simulink model "Demo919"  (R2018b)
settings: Solver=ode3  StartTime=0.0  StopTime=10  FixedStep=0.0005  RelTol=1e-3  EnableMultiTasking=on
values from neighbouring files (symbols this model uses):
  ADS1 = [1000 4000]    [data_new1.m]
  ADS2 = [900 4100]    [data_new1.m]
  br_opening = [0 20 40 60 80 100]    [data_new1.m]
  BRAKE = [485 1288 2091 2894 3697 4500]    [data_new1.m]
  InerWheel_Angle = [0 0.001 0.502 1.006 1.514 2.024 2.538 3.055 3.575 4.098 4.625 5.155 5.689 6.226 6.767 7.311 7.859 8.411 8.967 9.527 10.091 10.659 11.231 11.807 12.387 12.972 13.561 14.154 14.752 15.354 15.961 16.572 17.187 17.807 18.432 19.062 19.696 20.334 20.977 21.625 22.277 22.934 23.596 24.262 24.932 25.607 26.286 26.970 27.657 28.349 29.045 29.745 30.448 31.155 31.866]    [data_new1.m]
  OuterWheel_Angle = [0 0.001 0.501 1.001 1.501 2.001 2.501	3.001 3.501	4.001 4.501	5.001 5.501	6.001 6.501	7.001 7.501	8.001 8.501	9.001 9.501	10.001 10.501 11.001 11.501 12.001 12.501 13.001 13.501	14.001 14.501 15.001 15.501 16.001 16.501 17.001 17.501 18.001 18.501 19.001 19.501	20.001 20.501 21.001 21.501	22.001 22.501 23.001 23.501	24.001 24.501 25.001 25.501 26.001 26.501]    [data_new1.m]
  PUMP = [0 1000 2000 3000 4000 5000]    [data_new1.m]
  SteeringAngle_Cal = [-90 0 90]    [data_new1.m]
  SteeringAngle_Sensor = [640 1840 3041]    [data_new1.m]
  th_opening = [0 100]    [data_new1.m]
undefined symbols (not defined in the file or in its folder): D, I_AN06_5V, I_AN08_5V, I_AN09_5V, I_AN10_5V, I_HALL1, I_HALL2, I_SW01_L, I_SW10_L, I_SW11_H, I_SW12_H, I_SW13_H, I_SW14_H, I_SW15_H, I_SW16_H, I_SW17_H, I_SW18_H, I_SW19_H, I_SW20_H, O_PWM1_LS0A7, O_PWM2_LS0A7, O_SW02_LS0A4, O_SW13_HS1A, O_SW14_HS1A
libraries: ec5744lib x137, simulink x20, canmsglib x11
(part 2 of 5)

== system Demo919/Function-Call Subsystem1/Subsystem ==
  note: 油压范围在500到4500之间
  note: 输出12V高电平给蜂鸣器和待驶指示
      | 灯，启动鸣笛，指示灯亮
  Brake : Inport  OutDataTypeStr=uint16
  Key : Inport  Port=2
  MCU1_rdy : Inport  Port=3
  MCU2_rdy : Inport  Port=4
  DC_BusVoltH1 : Inport  Port=5
  DC_BusVoltL1 : Inport  Port=6
  DC_BusVoltH2 : Inport  Port=7
  DC_BusVoltL2 : Inport  Port=8
  1-D Lookup Table2 : Lookup_n-D  NumberOfTableDimensions=1  BreakpointsForDimension1=BRAKE  Table=br_opening  ExtrapMethod=Clip  InternalRulePriority=Speed  OutMin=0  OutMax=100  OutDataTypeStr=uint8  RndMeth=Simplest  InputSameDT=on
  MeaModule : ec5744lib/RapidECU_U3/07Calibration/MeaModule  signal=Wait_Start
      settings: SourceProductName=ECUCoder for MPC5744
  MeaModule1 : ec5744lib/RapidECU_U3/07Calibration/MeaModule  signal=Brake
      settings: SourceProductName=ECUCoder for MPC5744
  MeaModule2 : ec5744lib/RapidECU_U3/07Calibration/MeaModule  signal=brake
      settings: SourceProductName=ECUCoder for MPC5744
  MeaModule3 : ec5744lib/RapidECU_U3/07Calibration/MeaModule  signal=RS
      settings: SourceProductName=ECUCoder for MPC5744
  Subsystem1 : Subsystem
  Subsystem2 : Subsystem
  Terminator : Terminator
  WaitStart&Brake_LED : Stateflow chart  TreatAsAtomicUnit=on
  "Brake " : Outport
  Break_LED : Outport  Port=2
  WS_Sig : Outport  Port=3
  Wait_Start : Outport  Port=4
  wires:
  WaitStart&Brake_LED/1(Wait_Start) -> MeaModule/1  "Wait_Start"
  Brake/1 -> MeaModule2/1
  1-D Lookup Table2/1 -> "Brake "/1, MeaModule1/1
  WaitStart&Brake_LED/2(Break_LED) -> Break_LED/1  "Break_LED"
  Key/1 -> WaitStart&Brake_LED/2(Key)
  WaitStart&Brake_LED/3(WS_Sig) -> WS_Sig/1
  WaitStart&Brake_LED/4(RS) -> MeaModule3/1
  MeaModule3/1 -> Terminator/1
  MCU1_rdy/1 -> WaitStart&Brake_LED/3(MCU1_rdy)
  MCU2_rdy/1 -> WaitStart&Brake_LED/4(MCU2_rdy)
  MeaModule/1 -> Wait_Start/1
  DC_BusVoltH1/1 -> Subsystem1/1(DatH)
  DC_BusVoltL1/1 -> Subsystem1/2(DatL)
  DC_BusVoltH2/1 -> Subsystem2/1(DatH)
  DC_BusVoltL2/1 -> Subsystem2/2(DatL)
  Subsystem1/1(DC_BusVolt1) -> WaitStart&Brake_LED/5(DC_BusVolt1)
  Subsystem2/1(DC_BusVolt2) -> WaitStart&Brake_LED/6(DC_BusVolt2)
  MeaModule1/1 -> WaitStart&Brake_LED/1(Brake)
  MeaModule2/1 -> 1-D Lookup Table2/1

== system Demo919/Function-Call Subsystem1/Subsystem1 ==
  Re_Mot_Speed : Inport
  Add : Sum  AccumDataTypeStr=double
  Add1 : Sum  AccumDataTypeStr=double
  Add2 : Sum  Inputs=-+
  Add3 : Sum  Inputs=+-
  Bus Creator : BusCreator  Inputs=2
  Bus Selector : BusSelector  OutputSignals=Re_Mot_SpeedL1,Re_Mot_SpeedH1,Re_Mot_SpeedL2,Re_Mot_SpeedH2
  Constant : Constant  Value=10000
  Constant1 : Constant  Value=10000
  Data Type Conversion{,1..3} (4 alike) : DataTypeConversion  OutDataTypeStr=uint16
  Data Type Conversion6 : DataTypeConversion  OutDataTypeStr=double
  Data Type Conversion7 : DataTypeConversion  OutDataTypeStr=double
  Gain : Gain  Gain=0.5
  Gain1 : Gain  Gain=0.5
  Shift Arithmetic : ArithShift  BitShiftNumber=8  BitShiftDirection=Left
  Shift Arithmetic1 : ArithShift  BitShiftNumber=8  BitShiftDirection=Left
  Mot_Speed : Outport
  wires:
  Bus Selector/3 -> Data Type Conversion2/1  "<Re_Mot_SpeedL2>"
  Bus Selector/1 -> Data Type Conversion/1  "<Re_Mot_SpeedL1>"
  Bus Selector/2 -> Data Type Conversion1/1  "<Re_Mot_SpeedH1>"
  Re_Mot_Speed/1 -> Bus Selector/1
  Bus Selector/4 -> Data Type Conversion3/1  "<Re_Mot_SpeedH2>"
  Data Type Conversion6/1 -> Gain/1
  Data Type Conversion7/1 -> Gain1/1
  Constant1/1 -> Add3/2
  Constant/1 -> Add2/1
  Add3/1 -> Bus Creator/2
  Gain1/1 -> Add3/1
  Add2/1 -> Bus Creator/1
  Gain/1 -> Add2/2
  Bus Creator/1 -> Mot_Speed/1
  Data Type Conversion3/1 -> Shift Arithmetic1/1
  Add1/1 -> Data Type Conversion7/1
  Data Type Conversion2/1 -> Add1/1
  Shift Arithmetic1/1 -> Add1/2
  Add/1 -> Data Type Conversion6/1
  Shift Arithmetic/1 -> Add/2
  Data Type Conversion1/1 -> Shift Arithmetic/1
  Data Type Conversion/1 -> Add/1

== system Demo919/Function-Call Subsystem1/Subsystem2 ==
  Bus_Curr&Volt : Inport
  Abs : Abs
  Bus Selector6 : BusSelector  OutputSignals=Bat_Voltage_MSB,Bat_Voltage_LSB,Bat_Current_MSB,Bat_Current_LSB
  Gain : Gain  Gain=1/1000
  Product : Product
  Subsystem4 : Subsystem
  Subsystem5 : Subsystem
  P : Outport
  wires:
  Bus_Curr&Volt/1 -> Bus Selector6/1
  Gain/1 -> Abs/1
  Bus Selector6/1 -> Subsystem4/1(CurrH)  "<Bat_Voltage_MSB>"
  Bus Selector6/2 -> Subsystem4/2(CurrL)  "<Bat_Voltage_LSB>"
  Bus Selector6/3 -> Subsystem5/1(CurrH)  "<Bat_Current_MSB>"
  Bus Selector6/4 -> Subsystem5/2(CurrL)  "<Bat_Current_LSB>"
  Subsystem4/1(Bat_V) -> Product/1
  Subsystem5/1(Bat_A) -> Product/2
  Abs/1 -> P/1
  Product/1 -> Gain/1

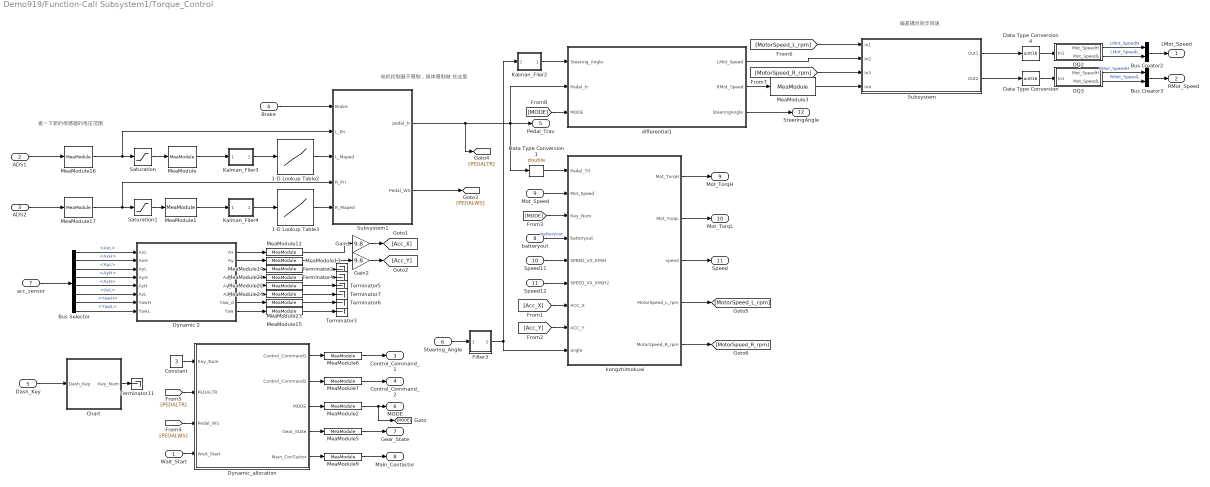
== system Demo919/Function-Call Subsystem1/Torque_Control ==
  note: 偏差耦合同步转速
  note: 查一下新的传感器的电压范围
  note: 电机控制器不限制，具体限制做
      | 在这里
  Wait_Start : Inport
  ADS1 : Inport  Port=2
  ADS2 : Inport  Port=3  OutDataTypeStr=uint16
  "Brake " : Inport  Port=4
  "Dash_Key " : Inport  Port=5  OutMin=0  OutMax=2
  Steering_Angle : Inport  Port=6
  acc_sensor : Inport  Port=7
  batteryout : Inport  Port=8
  Mot_Speed : Inport  Port=9
  Speed11 : Inport  Port=10
  Speed12 : Inport  Port=11
  1-D Lookup Table2 : Lookup_n-D  NumberOfTableDimensions=1  BreakpointsForDimension1=ADS1  Table=th_opening  ExtrapMethod=Clip  InternalRulePriority=Speed  OutMin=0  OutMax=95  OutDataTypeStr=double  RndMeth=Simplest  InputSameDT=on
  1-D Lookup Table3 : Lookup_n-D  NumberOfTableDimensions=1  BreakpointsForDimension1=ADS2  Table=th_opening  ExtrapMethod=Clip  InternalRulePriority=Speed  OutMin=0  OutMax=95  OutDataTypeStr=double  RndMeth=Simplest  InputSameDT=on
  Bus Creator2 : BusCreator  Inputs=2
  Bus Creator3 : BusCreator  Inputs=2
  Bus Selector : BusSelector  OutputSignals=AxL,AxH,AyL,AyH,AzH,AzL,YawH,YawL
  Chart : Stateflow chart  TreatAsAtomicUnit=on
  Constant : Constant  Value=3
  Data Type Conversion : DataTypeConversion  OutDataTypeStr=uint16
  Data Type Conversion1 : DataTypeConversion  OutDataTypeStr=double
  Data Type Conversion4 : DataTypeConversion  OutDataTypeStr=uint16
  Dynamic 2 : Stateflow chart  TreatAsAtomicUnit=on
  Dynamic_allocation : Stateflow chart  TreatAsAtomicUnit=on
  Filter3 : Subsystem
  Gain1 : Gain  Gain=9.8
  Gain2 : Gain  Gain=9.8
  Kalman_Filer2 : Subsystem
  Kalman_Filer3 : Subsystem
  Kalman_Filer4 : Subsystem
  MeaModule : ec5744lib/RapidECU_U3/07Calibration/MeaModule  signal=ADSH
      settings: SourceProductName=ECUCoder for MPC5744
  MeaModule1 : ec5744lib/RapidECU_U3/07Calibration/MeaModule  signal=ADSL
      settings: SourceProductName=ECUCoder for MPC5744
  MeaModule12 : ec5744lib/RapidECU_U3/07Calibration/MeaModule  signal=AX
      settings: SourceProductName=ECUCoder for MPC5744
  MeaModule13 : ec5744lib/RapidECU_U3/07Calibration/MeaModule  signal=AY
      settings: SourceProductName=ECUCoder for MPC5744
  MeaModule14 : ec5744lib/RapidECU_U3/07Calibration/MeaModule  signal=AZ
      settings: SourceProductName=ECUCoder for MPC5744
  MeaModule15 : ec5744lib/RapidECU_U3/07Calibration/MeaModule  signal=YAW
      settings: SourceProductName=ECUCoder for MPC5744
  MeaModule16 : ec5744lib/RapidECU_U3/07Calibration/MeaModule  signal=ADSh
      settings: SourceProductName=ECUCoder for MPC5744
  MeaModule17 : ec5744lib/RapidECU_U3/07Calibration/MeaModule  signal=ADSl
      settings: SourceProductName=ECUCoder for MPC5744
  MeaModule2 : ec5744lib/RapidECU_U3/07Calibration/MeaModule  signal=MODE
      settings: SourceProductName=ECUCoder for MPC5744
  MeaModule21 : ec5744lib/RapidECU_U3/07Calibration/MeaModule  signal=Ax_d
      settings: SourceProductName=ECUCoder for MPC5744
  MeaModule22 : ec5744lib/RapidECU_U3/07Calibration/MeaModule  signal=Ay_d
      settings: SourceProductName=ECUCoder for MPC5744
  MeaModule23 : ec5744lib/RapidECU_U3/07Calibration/MeaModule  signal=Yaw_d
      settings: SourceProductName=ECUCoder for MPC5744
  MeaModule24 : ec5744lib/RapidECU_U3/07Calibration/MeaModule  signal=Az_d
      settings: SourceProductName=ECUCoder for MPC5744
  MeaModule3 : ec5744lib/RapidECU_U3/07Calibration/MeaModule  signal=RMotSpeed
      settings: SourceProductName=ECUCoder for MPC5744
  MeaModule5 : ec5744lib/RapidECU_U3/07Calibration/MeaModule  signal=Gear_State
      settings: SourceProductName=ECUCoder for MPC5744
  MeaModule6 : ec5744lib/RapidECU_U3/07Calibration/MeaModule  signal=Control1
      settings: SourceProductName=ECUCoder for MPC5744
  MeaModule7 : ec5744lib/RapidECU_U3/07Calibration/MeaModule  signal=Control2
      settings: SourceProductName=ECUCoder for MPC5744
  MeaModule9 : ec5744lib/RapidECU_U3/07Calibration/MeaModule  signal=Main_Contactor
      settings: SourceProductName=ECUCoder for MPC5744
  OQ2 : Subsystem
  OQ3 : Subsystem
  Saturation : Saturate  UpperLimit=4000  LowerLimit=2000  OutDataTypeStr=double
  Saturation1 : Saturate  UpperLimit=3350  LowerLimit=1000  OutDataTypeStr=double
  Subsystem : Subsystem
  Subsystem1 : Subsystem
  Terminator{2..7,11} (7 alike) : Terminator
  differential1 : Subsystem
  kongzhimokuai : Subsystem
  LMot_Speed : Outport
  RMot_Speed : Outport  Port=2
  "Control_Command_1 " : Outport  Port=3  OutDataTypeStr=uint8
  Control_Command_2 : Outport  Port=4  OutDataTypeStr=uint8
  Pedal_Trav : Outport  Port=5
  MODE : Outport  Port=6
  "Gear_State " : Outport  Port=7
  Main_Contactor : Outport  Port=8
  Mot_TorqH : Outport  Port=9
  Mot_TorqL : Outport  Port=10
  Speed : Outport  Port=11
  SteeringAngle : Outport  Port=12
  wires:
  "Dash_Key "/1 -> Chart/1(Dash_Key)
  MeaModule1/1 -> Kalman_Filer4/1(In1)
  MeaModule6/1 -> "Control_Command_1 "/1
  MeaModule7/1 -> Control_Command_2/1
  Wait_Start/1 -> Dynamic_allocation/4(Wait_Start)
  MeaModule2/1 -> MODE/1, [MODE]
  MeaModule5/1 -> "Gear_State "/1
  MeaModule9/1 -> Main_Contactor/1
  acc_sensor/1 -> Bus Selector/1
  Dynamic 2/1(Ax) -> MeaModule12/1
  Dynamic 2/2(Ay) -> MeaModule13/1
  Dynamic 2/3(Az) -> MeaModule14/1
  MeaModule12/1 -> Gain1/1
  MeaModule13/1 -> Gain2/1
  MeaModule14/1 -> Terminator2/1
  MeaModule15/1 -> Terminator3/1
  Chart/1(Key_Num) -> Terminator11/1
  Subsystem1/1("pedal_tr ") -> [PEDALTR], Data Type Conversion1/1, Pedal_Trav/1, differential1/2(Pedal_tr)
  MeaModule21/1 -> Terminator4/1
  Dynamic 2/4(Ax_d) -> MeaModule21/1
  MeaModule22/1 -> Terminator5/1
  Dynamic 2/5(Ay_d) -> MeaModule22/1
  MeaModule23/1 -> Terminator6/1
  MeaModule24/1 -> Terminator7/1
  Dynamic 2/6(Az_d) -> MeaModule24/1
  Dynamic 2/7(Yaw_d) -> MeaModule23/1
  Dynamic 2/8(Yaw) -> MeaModule15/1
  Bus Selector/5 -> Dynamic 2/5(AzH)  "<AzH>"
  Bus Selector/6 -> Dynamic 2/6(AzL)  "<AzL>"
  Bus Selector/8 -> Dynamic 2/8(YawL)  "<YawL>"
  Bus Selector/7 -> Dynamic 2/7(YawH)  "<YawH>"
  Dynamic_allocation/1(Control_Command1) -> MeaModule6/1
  Dynamic_allocation/2(Control_Command2) -> MeaModule7/1
  Dynamic_allocation/3(MODE) -> MeaModule2/1
  Dynamic_allocation/4(Gear_State) -> MeaModule5/1
  Dynamic_allocation/5(Main_ConTactor) -> MeaModule9/1
  MeaModule16/1 -> Subsystem1/2(L_Pri), Saturation/1
  Saturation/1 -> MeaModule/1
  MeaModule17/1 -> Subsystem1/4(R_Pri), Saturation1/1
  Saturation1/1 -> MeaModule1/1
  Speed12/1 -> kongzhimokuai/6(SPEED_VX_KM/H2)
  batteryout/1 -> kongzhimokuai/4(batteryout)  "batteryout"
  Mot_Speed/1 -> kongzhimokuai/2(Mot_Speed)
  Speed11/1 -> kongzhimokuai/5(SPEED_VX_KM/H)
  Data Type Conversion1/1 -> kongzhimokuai/1(Pedal_Trl)
  "Brake "/1 -> Subsystem1/1("Brake ")
  kongzhimokuai/1(Mot_TorqH) -> Mot_TorqH/1
  kongzhimokuai/2(Mot_TorqL) -> Mot_TorqL/1
  [MODE] -> kongzhimokuai/3(Key_Num)
  1-D Lookup Table3/1 -> Subsystem1/5(R_Maped)
  Subsystem1/2("Pedal_WS ") -> [PEDALWS]
  [PEDALWS] -> Dynamic_allocation/3(Pedal_WS)
  Gain1/1 -> [Acc_X]
  Gain2/1 -> [Acc_Y]
  kongzhimokuai/3(speed) -> Speed/1
  [PEDALTR] -> Dynamic_allocation/2(PEDALTR)
  Constant/1 -> Dynamic_allocation/1(Key_Num)
  [Acc_X] -> kongzhimokuai/7(ACC_X)
  [Acc_Y] -> kongzhimokuai/8(ACC_Y)
  Bus Selector/1 -> Dynamic 2/1(AxL)  "<AxL>"
  Bus Selector/2 -> Dynamic 2/2(AxH)  "<AxH>"
  Bus Selector/3 -> Dynamic 2/3(AyL)  "<AyL>"
  Bus Selector/4 -> Dynamic 2/4(AyH)  "<AyH>"
  kongzhimokuai/4(MotorSpeed_L_rpm) -> [MotorSpeed_L_rpm]
  kongzhimokuai/5(MotorSpeed_R_rpm) -> [MotorSpeed_R_rpm]
  Data Type Conversion/1 -> OQ3/1(In1)
  Data Type Conversion4/1 -> OQ2/1(In1)
  differential1/3(SteeringAngle) -> SteeringAngle/1
  Bus Creator2/1 -> LMot_Speed/1
  OQ3/2(Mot_SpeedL) -> Bus Creator3/2  "RMot_SpeedL"
  Bus Creator3/1 -> RMot_Speed/1
  OQ2/2(Mot_SpeedL) -> Bus Creator2/2  "LMot_SpeedL"
  OQ3/1(Mot_SpeedH) -> Bus Creator3/1  "RMot_SpeedH"
  differential1/2(RMot_Speed) -> MeaModule3/1
  OQ2/1(Mot_SpeedH) -> Bus Creator2/1  "LMot_SpeedH"
  [MODE] -> differential1/3(MODE)
  MeaModule/1 -> Kalman_Filer3/1(In1)
  Steering_Angle/1 -> Filter3/1(In1)
  Kalman_Filer2/1(Out1) -> differential1/1(Steering_Angle)
  ADS1/1 -> MeaModule16/1
  ADS2/1 -> MeaModule17/1
  1-D Lookup Table2/1 -> Subsystem1/3(L_Maped)
  Kalman_Filer3/1(Out1) -> 1-D Lookup Table2/1
  Kalman_Filer4/1(Out1) -> 1-D Lookup Table3/1
  Filter3/1(Out1) -> kongzhimokuai/9(angle), Kalman_Filer2/1(In1)
  [MotorSpeed_L_rpm] -> Subsystem/1(In1)
  differential1/1(LMot_Speed) -> Subsystem/2(In2)
  [MotorSpeed_R_rpm] -> Subsystem/3(In3)
  MeaModule3/1 -> Subsystem/4(In4)
  Subsystem/1(Out1) -> Data Type Conversion4/1
  Subsystem/2(Out2) -> Data Type Conversion/1

== system Demo919/Function-Call Subsystem/Function-Call Subsystem/Enabled Subsystem ==
  note: 转化数据类型也许可以把内存降到更低，但是我觉得这个就是后话了[doge]
  In1 : Inport
  In2 : Inport  Port=2
  Enable : EnablePort
  CAN Unpack : canmsglib/CAN Unpack  CANdbFile=E:\project\DBC_file\MotControl.dbc  MsgList=BMStoVCU_1  MsgName=BMStoVCU_1  MsgIDType=Extended (29-bit identifier)  MsgIdentifier=408961267  MsgLength=8  SignalInfo=BatAlmLv$52$4$1$2$1$0$1$0$0$15$#BatCurrent_LSB$24$8$1$2$1$0$1$0$0$255$#BatCurrent_MSB$16$8$1$2$1$0$1$0$0$255$#BatLife$56$8$1$2$1$0$1$0$0$255$#BatSoc$32$8$1$2$1$0$1$0$0$255$#BatSoh$40$8$1$2$1$0$1$0$0$255$#BatState$48$4$1$2$1$0$1$0$0$15$#BatVoltage_LSB$8$8$1$2$1$0$1$0$0$255$#BatVoltage_MSB$0$8$1$2$1$0$1$0$0$255$#  NSignals=9  IDPort=off  TimestampPort=off  ErrorPort=off  RemotePort=off  LengthPort=off  StatusPort=off  StartBits=str2num('[int32(52);int32(24);int32(16);int32(56);int32(32);int32(40);int32(48);int32(8);int32(0)]')  SignalSizes=str2num('[int32(4);int32(8);int32(8);int32(8);int32(8);int32(8);int32(4);int32(8);int32(8)]')  ByteOrders=str2num('[int32(1);int32(1);int32(1);int32(1);int32(1);int32(1);int32(1);int32(1);int32(1)]')  DataTypes=str2num('[int32(2);int32(2);int32(2);int32(2);int32(2);int32(2);int32(2);int32(2);int32(2)]')  MultiplexTypes=str2num('[int32(1);int32(1);int32(1);int32(1);int32(1);int32(1);int32(1);int32(1);int32(1)]')  MultiplexValues=str2num('[double(0);double(0);double(0);double(0);double(0);double(0);double(0);double(0);double(0)]')  Factors=str2num('[double(1);double(1);double(1);double(1);double(1);double(1);double(1);double(1);double(1)]')  Offsets=str2num('[double(0);double(0);double(0);double(0);double(0);double(0);double(0);double(0);double(0)]')  Minimums=str2num('[double(0);double(0);double(0);double(0);double(0);double(0);double(0);double(0);double(0)]')  Maximums=str2num('[double(15);double(255);double(255);double(255);double(255);double(255);double(15);double(255);double(255)]')  ApplyMinMax=off
      settings: SourceProductName=Simulink Real-Time  SourceProductBaseCode=XP  DataFormat=CANdb specified signals
  CANUnPackMessage : ec5744lib/RapidECU_U3/04CANCommunication/CANUnPackMessage  datalength=8  canmessagetype=Extended(29-bit ID)  sampletime=-1
      settings: SourceProductName=ECUCoder for MPC5744
  "Bat_Voltage_LSB " : Outport
  Bat_Current_MSB : Outport  Port=2
  "BatAlmLv " : Outport  Port=3
  BatLife : Outport  Port=4
  BatSoc : Outport  Port=5
  BatSoh : Outport  Port=6
  BatState : Outport  Port=7
  Bat_Current_LSB : Outport  Port=8
  "Bat_Voltage_MSB " : Outport  Port=9
  wires:
  CANUnPackMessage/1 -> CAN Unpack/1
  In2/1 -> CANUnPackMessage/2
  In1/1 -> CANUnPackMessage/1
  CAN Unpack/8 -> "Bat_Voltage_LSB "/1
  CAN Unpack/9 -> "Bat_Voltage_MSB "/1
  CAN Unpack/3 -> Bat_Current_MSB/1
  CAN Unpack/1 -> "BatAlmLv "/1
  CAN Unpack/5 -> BatSoc/1
  CAN Unpack/6 -> BatSoh/1
  CAN Unpack/7 -> BatState/1
  CAN Unpack/2 -> Bat_Current_LSB/1
  CAN Unpack/4 -> BatLife/1

== system Demo919/Function-Call Subsystem/Function-Call Subsystem1/Enabled Subsystem ==
  note: 转化数据类型也许可以把内存降到更低，但是我觉得这个就是后话了[doge]
  In1 : Inport
  In2 : Inport  Port=2
  Enable : EnablePort
  CAN Unpack : canmsglib/CAN Unpack  CANdbFile=E:\project\DBC_file\MotControl.dbc  MsgList=MCU1toVCU_1  MsgName=MCU1toVCU_1  MsgIDType=Extended (29-bit identifier)  MsgIdentifier=218089199  MsgLength=8  SignalInfo=Com_Alarm1$56$2$1$2$1$0$1$0$0$3$#ControlMode_Command1$32$8$1$2$1$0$1$0$0$255$#MCU1State1$40$8$1$2$1$0$1$0$0$255$#MCU1State2$48$2$1$2$1$0$1$0$0$3$#Re_Mot_SpeedH1$8$8$1$2$1$0$1$0$0$255$#Re_Mot_SpeedL1$0$8$1$2$1$0$1$0$0$255$#Re_Mot_TorqueH1$24$8$1$2$1$0$1$0$0$255$#Re_Mot_TorqueL1$16$8$1$2$1$0$1$0$0$255$#Self_Test1$55$1$1$2$1$0$1$0$0$1$#  NSignals=9  IDPort=off  TimestampPort=off  ErrorPort=off  RemotePort=off  LengthPort=off  StatusPort=off  StartBits=str2num('[int32(56);int32(32);int32(40);int32(48);int32(8);int32(0);int32(24);int32(16);int32(55)]')  SignalSizes=str2num('[int32(2);int32(8);int32(8);int32(2);int32(8);int32(8);int32(8);int32(8);int32(1)]')  ByteOrders=str2num('[int32(1);int32(1);int32(1);int32(1);int32(1);int32(1);int32(1);int32(1);int32(1)]')  DataTypes=str2num('[int32(2);int32(2);int32(2);int32(2);int32(2);int32(2);int32(2);int32(2);int32(2)]')  MultiplexTypes=str2num('[int32(1);int32(1);int32(1);int32(1);int32(1);int32(1);int32(1);int32(1);int32(1)]')  MultiplexValues=str2num('[double(0);double(0);double(0);double(0);double(0);double(0);double(0);double(0);double(0)]')  Factors=str2num('[double(1);double(1);double(1);double(1);double(1);double(1);double(1);double(1);double(1)]')  Offsets=str2num('[double(0);double(0);double(0);double(0);double(0);double(0);double(0);double(0);double(0)]')  Minimums=str2num('[double(0);double(0);double(0);double(0);double(0);double(0);double(0);double(0);double(0)]')  Maximums=str2num('[double(3);double(255);double(255);double(3);double(255);double(255);double(255);double(255);double(1)]')  ApplyMinMax=off
      settings: SourceProductName=Simulink Real-Time  SourceProductBaseCode=XP  DataFormat=CANdb specified signals
  CANUnPackMessage : ec5744lib/RapidECU_U3/04CANCommunication/CANUnPackMessage  datalength=8  canmessagetype=Extended(29-bit ID)  sampletime=-1
      settings: SourceProductName=ECUCoder for MPC5744
  Terminator{,1,3..4} (4 alike) : Terminator
  Pe_Mot_SpeedH1 : Outport
  Re_MotSpeedL1 : Outport  Port=2
  Re_Mot_TorqueH1 : Outport  Port=3
  Re_MotTorqueL1 : Outport  Port=4
  MCU1State1 : Outport  Port=5
  wires:
  CAN Unpack/4 -> Terminator3/1
  CAN Unpack/2 -> Terminator1/1
  CAN Unpack/7 -> Re_Mot_TorqueH1/1
  CAN Unpack/6 -> Re_MotSpeedL1/1
  CAN Unpack/5 -> Pe_Mot_SpeedH1/1
  CAN Unpack/1 -> Terminator/1
  CAN Unpack/3 -> MCU1State1/1
  CAN Unpack/9 -> Terminator4/1
  CAN Unpack/8 -> Re_MotTorqueL1/1
  In1/1 -> CANUnPackMessage/1
  In2/1 -> CANUnPackMessage/2
  CANUnPackMessage/1 -> CAN Unpack/1

== system Demo919/Function-Call Subsystem/Function-Call Subsystem2/Enabled Subsystem ==
  In1 : Inport
  In2 : Inport  Port=2
  Enable : EnablePort
  CAN Unpack : canmsglib/CAN Unpack  CANdbFile=E:\project\DBC_file\MotControl.dbc  MsgList=acc1  MsgName=acc1  MsgIDType=Standard (11-bit identifier)  MsgIdentifier=343  MsgLength=8  SignalInfo=PitchH$8$8$1$2$1$0$1$0$0$255$#PitchL$0$8$1$2$1$0$1$0$0$255$#RollH$24$8$1$2$1$0$1$0$0$255$#RollL$16$8$1$2$1$0$1$0$0$255$#  NSignals=4  IDPort=off  TimestampPort=off  ErrorPort=off  RemotePort=off  LengthPort=off  StatusPort=off  StartBits=str2num('[int32(8);int32(0);int32(24);int32(16)]')  SignalSizes=str2num('[int32(8);int32(8);int32(8);int32(8)]')  ByteOrders=str2num('[int32(1);int32(1);int32(1);int32(1)]')  DataTypes=str2num('[int32(2);int32(2);int32(2);int32(2)]')  MultiplexTypes=str2num('[int32(1);int32(1);int32(1);int32(1)]')  MultiplexValues=str2num('[double(0);double(0);double(0);double(0)]')  Factors=str2num('[double(1);double(1);double(1);double(1)]')  Offsets=str2num('[double(0);double(0);double(0);double(0)]')  Minimums=str2num('[double(0);double(0);double(0);double(0)]')  Maximums=str2num('[double(255);double(255);double(255);double(255)]')  ApplyMinMax=off
      settings: SourceProductName=Simulink Real-Time  SourceProductBaseCode=XP  DataFormat=CANdb specified signals
  CANUnPackMessage : ec5744lib/RapidECU_U3/04CANCommunication/CANUnPackMessage  datalength=8  canmessagetype=Standard(11-bit ID)  sampletime=-1
      settings: SourceProductName=ECUCoder for MPC5744
  PitchH : Outport
  PitchL : Outport  Port=2
  RollH : Outport  Port=3
  RollL : Outport  Port=4
  wires:
  CANUnPackMessage/1 -> CAN Unpack/1
  In2/1 -> CANUnPackMessage/2
  In1/1 -> CANUnPackMessage/1
  CAN Unpack/1 -> PitchH/1
  CAN Unpack/2 -> PitchL/1
  CAN Unpack/3 -> RollH/1
  CAN Unpack/4 -> RollL/1

== system Demo919/Function-Call Subsystem/Function-Call Subsystem3/Enabled Subsystem ==
  In1 : Inport
  In2 : Inport  Port=2
  Enable : EnablePort
  CAN Unpack : canmsglib/CAN Unpack  CANdbFile=E:\project\DBC_file\MotControl.dbc  MsgList=MCU2toVCU_1  MsgName=MCU2toVCU_1  MsgIDType=Extended (29-bit identifier)  MsgIdentifier=213000687  MsgLength=8  SignalInfo=Com_Alarm2$56$2$1$2$1$0$1$0$0$3$#ControlMode_Command2$32$8$1$2$1$0$1$0$0$255$#MCU2State1$40$8$1$2$1$0$1$0$0$255$#MCU2State2$48$2$1$2$1$0$1$0$0$3$#Re_Mot_SpeedH2$8$8$1$2$1$0$1$0$0$255$#Re_Mot_SpeedL2$0$8$1$2$1$0$1$0$0$255$#Re_Mot_TorqueH2$24$8$1$2$1$0$1$0$0$255$#Re_Mot_TorqueL2$16$8$1$2$1$0$1$0$0$255$#Selt_Test2$55$1$1$2$1$0$1$0$0$1$#  NSignals=9  IDPort=off  TimestampPort=off  ErrorPort=off  RemotePort=off  LengthPort=off  StatusPort=off  StartBits=str2num('[int32(56);int32(32);int32(40);int32(48);int32(8);int32(0);int32(24);int32(16);int32(55)]')  SignalSizes=str2num('[int32(2);int32(8);int32(8);int32(2);int32(8);int32(8);int32(8);int32(8);int32(1)]')  ByteOrders=str2num('[int32(1);int32(1);int32(1);int32(1);int32(1);int32(1);int32(1);int32(1);int32(1)]')  DataTypes=str2num('[int32(2);int32(2);int32(2);int32(2);int32(2);int32(2);int32(2);int32(2);int32(2)]')  MultiplexTypes=str2num('[int32(1);int32(1);int32(1);int32(1);int32(1);int32(1);int32(1);int32(1);int32(1)]')  MultiplexValues=str2num('[double(0);double(0);double(0);double(0);double(0);double(0);double(0);double(0);double(0)]')  Factors=str2num('[double(1);double(1);double(1);double(1);double(1);double(1);double(1);double(1);double(1)]')  Offsets=str2num('[double(0);double(0);double(0);double(0);double(0);double(0);double(0);double(0);double(0)]')  Minimums=str2num('[double(0);double(0);double(0);double(0);double(0);double(0);double(0);double(0);double(0)]')  Maximums=str2num('[double(3);double(255);double(255);double(3);double(255);double(255);double(255);double(255);double(1)]')  ApplyMinMax=off
      settings: SourceProductName=Simulink Real-Time  SourceProductBaseCode=XP  DataFormat=CANdb specified signals
  CANUnPackMessage : ec5744lib/RapidECU_U3/04CANCommunication/CANUnPackMessage  datalength=8  canmessagetype=Extended(29-bit ID)  sampletime=-1
      settings: SourceProductName=ECUCoder for MPC5744
  Terminator{,1,3..4} (4 alike) : Terminator
  Re_Mot_SpeedH2 : Outport
  Re_Mot_SpeedL2 : Outport  Port=2
  Re_Mot_TorqueH2 : Outport  Port=3
  Re_Mot_TorqueL2 : Outport  Port=4
  MCU2State1 : Outport  Port=5
  wires:
  In1/1 -> CANUnPackMessage/1
  In2/1 -> CANUnPackMessage/2
  CANUnPackMessage/1 -> CAN Unpack/1
  CAN Unpack/7 -> Re_Mot_TorqueH2/1
  CAN Unpack/4 -> Terminator3/1
  CAN Unpack/6 -> Re_Mot_SpeedL2/1
  CAN Unpack/2 -> Terminator1/1
  CAN Unpack/9 -> Terminator4/1
  CAN Unpack/5 -> Re_Mot_SpeedH2/1
  CAN Unpack/3 -> MCU2State1/1
  CAN Unpack/8 -> Re_Mot_TorqueL2/1
  CAN Unpack/1 -> Terminator/1

== system Demo919/Function-Call Subsystem/Function-Call Subsystem4/Enabled Subsystem ==
  In1 : Inport
  In2 : Inport  Port=2
  Enable : EnablePort
  CAN Unpack : canmsglib/CAN Unpack  CANdbFile=E:\project\DBC_file\MotControl.dbc  MsgList=MCU1toVCU_2  MsgName=MCU1toVCU_2  MsgIDType=Extended (29-bit identifier)  MsgIdentifier=218089455  MsgLength=8  SignalInfo=AC_CurValidH1$56$8$1$2$1$0$1$0$0$255$#AC_CurValidL1$48$8$1$2$1$0$1$0$0$255$#DC_Bus_CurrH1$40$8$1$2$1$0$1$0$0$255$#DC_Bus_CurrL1$32$8$1$2$1$0$1$0$0$255$#DC_Bus_VoltH1$24$8$1$2$1$0$1$0$0$255$#DC_Bus_VoltL1$16$8$1$2$1$0$1$0$0$255$#MotControllerTem1$0$8$1$2$1$0$1$0$0$255$#Mot_Tem1$8$8$1$2$1$0$1$0$0$255$#  NSignals=8  IDPort=off  TimestampPort=off  ErrorPort=off  RemotePort=off  LengthPort=off  StatusPort=off  StartBits=str2num('[int32(56);int32(48);int32(40);int32(32);int32(24);int32(16);int32(0);int32(8)]')  SignalSizes=str2num('[int32(8);int32(8);int32(8);int32(8);int32(8);int32(8);int32(8);int32(8)]')  ByteOrders=str2num('[int32(1);int32(1);int32(1);int32(1);int32(1);int32(1);int32(1);int32(1)]')  DataTypes=str2num('[int32(2);int32(2);int32(2);int32(2);int32(2);int32(2);int32(2);int32(2)]')  MultiplexTypes=str2num('[int32(1);int32(1);int32(1);int32(1);int32(1);int32(1);int32(1);int32(1)]')  MultiplexValues=str2num('[double(0);double(0);double(0);double(0);double(0);double(0);double(0);double(0)]')  Factors=str2num('[double(1);double(1);double(1);double(1);double(1);double(1);double(1);double(1)]')  Offsets=str2num('[double(0);double(0);double(0);double(0);double(0);double(0);double(0);double(0)]')  Minimums=str2num('[double(0);double(0);double(0);double(0);double(0);double(0);double(0);double(0)]')  Maximums=str2num('[double(255);double(255);double(255);double(255);double(255);double(255);double(255);double(255)]')  ApplyMinMax=off
      settings: SourceProductName=Simulink Real-Time  SourceProductBaseCode=XP  DataFormat=CANdb specified signals
  CANUnPackMessage : ec5744lib/RapidECU_U3/04CANCommunication/CANUnPackMessage  datalength=8  canmessagetype=Extended(29-bit ID)  sampletime=-1
      settings: SourceProductName=ECUCoder for MPC5744
  Terminator : Terminator
  Terminator1 : Terminator
  MotControllerTem1 : Outport
  Mot_Tem1 : Outport  Port=2
  DC_Bus_VoltH1 : Outport  Port=3
  DC_Bus_VoltL1 : Outport  Port=4
  DC_Bus_CurrH1 : Outport  Port=5
  DC_Bus_CurrL1 : Outport  Port=6
  wires:
  CANUnPackMessage/1 -> CAN Unpack/1
  In2/1 -> CANUnPackMessage/2
  In1/1 -> CANUnPackMessage/1
  CAN Unpack/1 -> Terminator/1
  CAN Unpack/3 -> DC_Bus_CurrH1/1
  CAN Unpack/2 -> Terminator1/1
  CAN Unpack/5 -> DC_Bus_VoltH1/1
  CAN Unpack/6 -> DC_Bus_VoltL1/1
  CAN Unpack/4 -> DC_Bus_CurrL1/1
  CAN Unpack/7 -> MotControllerTem1/1
  CAN Unpack/8 -> Mot_Tem1/1

== system Demo919/Function-Call Subsystem/Function-Call Subsystem6/Enabled Subsystem ==
  In1 : Inport
  In2 : Inport  Port=2
  Enable : EnablePort
  CAN Unpack : canmsglib/CAN Unpack  CANdbFile=E:\project\DBC_file\MotControl.dbc  MsgList=DashtoVCU  MsgName=DashtoVCU  MsgIDType=Standard (11-bit identifier)  MsgIdentifier=341  MsgLength=8  SignalInfo=Dash_Key$0$8$1$2$1$0$1$0$0$255$#  NSignals=1  IDPort=off  TimestampPort=off  ErrorPort=off  RemotePort=off  LengthPort=off  StatusPort=off  StartBits=str2num('[int32(0)]')  SignalSizes=str2num('[int32(8)]')  ByteOrders=str2num('[int32(1)]')  DataTypes=str2num('[int32(2)]')  MultiplexTypes=str2num('[int32(1)]')  MultiplexValues=str2num('[double(0)]')  Factors=str2num('[double(1)]')  Offsets=str2num('[double(0)]')  Minimums=str2num('[double(0)]')  Maximums=str2num('[double(255)]')  ApplyMinMax=off
      settings: SourceProductName=Simulink Real-Time  SourceProductBaseCode=XP  DataFormat=CANdb specified signals
  CANUnPackMessage : ec5744lib/RapidECU_U3/04CANCommunication/CANUnPackMessage  datalength=8  canmessagetype=Standard(11-bit ID)  sampletime=-1
      settings: SourceProductName=ECUCoder for MPC5744
  Out1 : Outport
  wires:
  CANUnPackMessage/1 -> CAN Unpack/1
  In2/1 -> CANUnPackMessage/2
  In1/1 -> CANUnPackMessage/1
  CAN Unpack/1 -> Out1/1

== system Demo919/Function-Call Subsystem/Function-Call Subsystem7/Enabled Subsystem ==
  In1 : Inport
  In2 : Inport  Port=2
  Enable : EnablePort
  CAN Unpack : canmsglib/CAN Unpack  CANdbFile=E:\project\DBC_file\MotControl.dbc  MsgList=acc  MsgName=acc  MsgIDType=Standard (11-bit identifier)  MsgIdentifier=342  MsgLength=8  SignalInfo=AxH$8$8$1$2$1$0$1$0$0$255$#AxL$0$8$1$2$1$0$1$0$0$255$#AyH$24$8$1$2$1$0$1$0$0$255$#AyL$16$8$1$2$1$0$1$0$0$255$#AzH$40$8$1$2$1$0$1$0$0$255$#AzL$32$8$1$2$1$0$1$0$0$255$#YawH$56$8$1$2$1$0$1$0$0$255$#YawL$48$8$1$2$1$0$1$0$0$255$#  NSignals=8  IDPort=off  TimestampPort=off  ErrorPort=off  RemotePort=off  LengthPort=off  StatusPort=off  StartBits=str2num('[int32(8);int32(0);int32(24);int32(16);int32(40);int32(32);int32(56);int32(48)]')  SignalSizes=str2num('[int32(8);int32(8);int32(8);int32(8);int32(8);int32(8);int32(8);int32(8)]')  ByteOrders=str2num('[int32(1);int32(1);int32(1);int32(1);int32(1);int32(1);int32(1);int32(1)]')  DataTypes=str2num('[int32(2);int32(2);int32(2);int32(2);int32(2);int32(2);int32(2);int32(2)]')  MultiplexTypes=str2num('[int32(1);int32(1);int32(1);int32(1);int32(1);int32(1);int32(1);int32(1)]')  MultiplexValues=str2num('[double(0);double(0);double(0);double(0);double(0);double(0);double(0);double(0)]')  Factors=str2num('[double(1);double(1);double(1);double(1);double(1);double(1);double(1);double(1)]')  Offsets=str2num('[double(0);double(0);double(0);double(0);double(0);double(0);double(0);double(0)]')  Minimums=str2num('[double(0);double(0);double(0);double(0);double(0);double(0);double(0);double(0)]')  Maximums=str2num('[double(255);double(255);double(255);double(255);double(255);double(255);double(255);double(255)]')  ApplyMinMax=off
      settings: SourceProductName=Simulink Real-Time  SourceProductBaseCode=XP  DataFormat=CANdb specified signals
  CANUnPackMessage : ec5744lib/RapidECU_U3/04CANCommunication/CANUnPackMessage  datalength=8  canmessagetype=Standard(11-bit ID)  sampletime=-1
      settings: SourceProductName=ECUCoder for MPC5744
  AxH : Outport
  AXL : Outport  Port=2
  AyH : Outport  Port=3
  AyL : Outport  Port=4
  AzH : Outport  Port=5
  AzL : Outport  Port=6
  YawH : Outport  Port=7
  YawL : Outport  Port=8
  wires:
  CANUnPackMessage/1 -> CAN Unpack/1
  In2/1 -> CANUnPackMessage/2
  In1/1 -> CANUnPackMessage/1
  CAN Unpack/1 -> AxH/1
  CAN Unpack/2 -> AXL/1
  CAN Unpack/3 -> AyH/1
  CAN Unpack/4 -> AyL/1
  CAN Unpack/5 -> AzH/1
  CAN Unpack/6 -> AzL/1
  CAN Unpack/7 -> YawH/1
  CAN Unpack/8 -> YawL/1

== system Demo919/Function-Call Subsystem/Function-Call Subsystem8/Enabled Subsystem ==
  In1 : Inport
  In2 : Inport  Port=2
  Enable : EnablePort
  CAN Unpack : canmsglib/CAN Unpack  CANdbFile=E:\project\DBC_file\MotControl.dbc  MsgList=MCU2toVCU_2  MsgName=MCU2toVCU_2  MsgIDType=Extended (29-bit identifier)  MsgIdentifier=213066223  MsgLength=8  SignalInfo=AC_CurValidH2$56$8$1$2$1$0$1$0$0$255$#AC_CurValidL2$48$8$1$2$1$0$1$0$0$255$#DC_Bus_CurrH2$40$8$1$2$1$0$1$0$0$255$#DC_Bus_CurrL2$32$8$1$2$1$0$1$0$0$255$#DC_Bus_VoltH2$24$8$1$2$1$0$1$0$0$255$#DC_Bus_VoltL2$16$8$1$2$1$0$1$0$0$255$#MotControllerTem2$0$8$1$2$1$0$1$0$0$255$#Mot_Tem2$8$8$1$2$1$0$1$0$0$255$#  NSignals=8  IDPort=off  TimestampPort=off  ErrorPort=off  RemotePort=off  LengthPort=off  StatusPort=off  StartBits=str2num('[int32(56);int32(48);int32(40);int32(32);int32(24);int32(16);int32(0);int32(8)]')  SignalSizes=str2num('[int32(8);int32(8);int32(8);int32(8);int32(8);int32(8);int32(8);int32(8)]')  ByteOrders=str2num('[int32(1);int32(1);int32(1);int32(1);int32(1);int32(1);int32(1);int32(1)]')  DataTypes=str2num('[int32(2);int32(2);int32(2);int32(2);int32(2);int32(2);int32(2);int32(2)]')  MultiplexTypes=str2num('[int32(1);int32(1);int32(1);int32(1);int32(1);int32(1);int32(1);int32(1)]')  MultiplexValues=str2num('[double(0);double(0);double(0);double(0);double(0);double(0);double(0);double(0)]')  Factors=str2num('[double(1);double(1);double(1);double(1);double(1);double(1);double(1);double(1)]')  Offsets=str2num('[double(0);double(0);double(0);double(0);double(0);double(0);double(0);double(0)]')  Minimums=str2num('[double(0);double(0);double(0);double(0);double(0);double(0);double(0);double(0)]')  Maximums=str2num('[double(255);double(255);double(255);double(255);double(255);double(255);double(255);double(255)]')  ApplyMinMax=off
      settings: SourceProductName=Simulink Real-Time  SourceProductBaseCode=XP  DataFormat=CANdb specified signals
  CANUnPackMessage : ec5744lib/RapidECU_U3/04CANCommunication/CANUnPackMessage  datalength=8  canmessagetype=Extended(29-bit ID)  sampletime=-1
      settings: SourceProductName=ECUCoder for MPC5744
  Terminator : Terminator
  Terminator1 : Terminator
  MotControllerTem2 : Outport
  Mot_Tem2 : Outport  Port=2
  DC_BusVoltH2 : Outport  Port=3
  DC_BusVoltL2 : Outport  Port=4
  DC_Bus_CurrH1 : Outport  Port=5
  DC_Bus_CurrL1 : Outport  Port=6
  wires:
  CANUnPackMessage/1 -> CAN Unpack/1
  In2/1 -> CANUnPackMessage/2
  In1/1 -> CANUnPackMessage/1
  CAN Unpack/3 -> DC_Bus_CurrH1/1
  CAN Unpack/1 -> Terminator/1
  CAN Unpack/2 -> Terminator1/1
  CAN Unpack/7 -> MotControllerTem2/1
  CAN Unpack/8 -> Mot_Tem2/1
  CAN Unpack/5 -> DC_BusVoltH2/1
  CAN Unpack/4 -> DC_Bus_CurrL1/1
  CAN Unpack/6 -> DC_BusVoltL2/1

== system Demo919/Function-Call Subsystem1/Subsystem/Subsystem1 ==
  DatH : Inport
  DatL : Inport  Port=2
  Chart : Stateflow chart  TreatAsAtomicUnit=on
  Data Type Conversion : DataTypeConversion  OutDataTypeStr=uint16
  Data Type Conversion1 : DataTypeConversion  OutDataTypeStr=uint16
  MeaModule1 : ec5744lib/RapidECU_U3/07Calibration/MeaModule  signal=DC_Bus1
      settings: SourceProductName=ECUCoder for MPC5744
  DC_BusVolt1 : Outport
  wires:
  DatL/1 -> Data Type Conversion/1
  DatH/1 -> Data Type Conversion1/1
  Data Type Conversion/1 -> Chart/2(DC_Bus_VoltL1)
  Data Type Conversion1/1 -> Chart/1(DC_Bus_VoltH1)
  Chart/1(DC_BusVolt1) -> MeaModule1/1
  MeaModule1/1 -> DC_BusVolt1/1

== system Demo919/Function-Call Subsystem1/Subsystem/Subsystem2 ==
  DatH : Inport
  DatL : Inport  Port=2
  Chart : Stateflow chart  TreatAsAtomicUnit=on
  Data Type Conversion : DataTypeConversion  OutDataTypeStr=uint16
  Data Type Conversion1 : DataTypeConversion  OutDataTypeStr=uint16
  MeaModule1 : ec5744lib/RapidECU_U3/07Calibration/MeaModule  signal=DC_Bus2
      settings: SourceProductName=ECUCoder for MPC5744
  DC_BusVolt2 : Outport
  wires:
  DatL/1 -> Data Type Conversion/1
  DatH/1 -> Data Type Conversion1/1
  Data Type Conversion/1 -> Chart/2(DC_Bus_VoltL1)
  Data Type Conversion1/1 -> Chart/1(DC_Bus_VoltH1)
  Chart/1(DC_BusVolt1) -> MeaModule1/1
  MeaModule1/1 -> DC_BusVolt2/1

== system Demo919/Function-Call Subsystem1/Subsystem2/Subsystem4 ==
  CurrH : Inport
  CurrL : Inport  Port=2
  Add : Sum  AccumDataTypeStr=double
  Data Type Conversion : DataTypeConversion  OutDataTypeStr=uint16
  Data Type Conversion1 : DataTypeConversion  OutDataTypeStr=uint16
  Data Type Conversion6 : DataTypeConversion  OutDataTypeStr=double
  Gain : Gain  Gain=0.1
  MeaModule1 : ec5744lib/RapidECU_U3/07Calibration/MeaModule  signal=Bat_V
      settings: SourceProductName=ECUCoder for MPC5744
  Shift Arithmetic : ArithShift  BitShiftNumber=8  BitShiftDirection=Left
  Bat_V : Outport
  wires:
  Data Type Conversion1/1 -> Add/2
  Shift Arithmetic/1 -> Add/1
  Data Type Conversion/1 -> Shift Arithmetic/1
  MeaModule1/1 -> Bat_V/1
  Data Type Conversion6/1 -> Gain/1
  CurrH/1 -> Data Type Conversion/1
  Gain/1 -> MeaModule1/1
  Add/1 -> Data Type Conversion6/1
  CurrL/1 -> Data Type Conversion1/1

== system Demo919/Function-Call Subsystem1/Subsystem2/Subsystem5 ==
  CurrH : Inport
  CurrL : Inport  Port=2
  Add : Sum  AccumDataTypeStr=double
  Add1 : Sum  Inputs=+-
  Constant : Constant  Value=1000
  Data Type Conversion : DataTypeConversion  OutDataTypeStr=uint16
  Data Type Conversion1 : DataTypeConversion  OutDataTypeStr=uint16
  Data Type Conversion6 : DataTypeConversion  OutDataTypeStr=double
  Gain : Gain  Gain=0.1
  MeaModule1 : ec5744lib/RapidECU_U3/07Calibration/MeaModule  signal=Bat_A
      settings: SourceProductName=ECUCoder for MPC5744
  Shift Arithmetic : ArithShift  BitShiftNumber=8  BitShiftDirection=Left
  Bat_A : Outport
  wires:
  CurrL/1 -> Data Type Conversion1/1
  Add/1 -> Data Type Conversion6/1
  CurrH/1 -> Data Type Conversion/1
  Data Type Conversion6/1 -> Gain/1
  MeaModule1/1 -> Bat_A/1
  Data Type Conversion/1 -> Shift Arithmetic/1
  Shift Arithmetic/1 -> Add/1
  Data Type Conversion1/1 -> Add/2
  Gain/1 -> Add1/1
  Add1/1 -> MeaModule1/1
  Constant/1 -> Add1/2

== system Demo919/Function-Call Subsystem1/Torque_Control/Filter3 ==
  note: 均值滤波器
  In1 : Inport
  Add2 : Sum  Inputs=-+-
  Gain2 : Gain  Gain=1/4
  MinMax : MinMax
  MinMax1 : MinMax  Function=max
  Sum of Elements : Sum  Inputs=+
  Tapped Delay : simulink/Discrete/Tapped Delay  vinit=0.0  samptime=-1  NumDelays=6  DelayOrder=Oldest  includeCurrent=off
  Out1 : Outport
  wires:
  In1/1 -> Tapped Delay/1
  Add2/1 -> Gain2/1
  MinMax/1 -> Add2/3
  MinMax1/1 -> Add2/1
  Gain2/1 -> Out1/1
  Sum of Elements/1 -> Add2/2
  Tapped Delay/1 -> MinMax/1, MinMax1/1, Sum of Elements/1

== system Demo919/Function-Call Subsystem1/Torque_Control/Kalman_Filer2 ==
  In1 : Inport
  Data Type Conversion : DataTypeConversion  OutDataTypeStr=single
  Data Type Conversion1 : DataTypeConversion  OutDataTypeStr=single
  Delay : Delay  DelayLength=1  InitialCondition=0
  Delay1 : Delay  DelayLength=1  InitialCondition=0
  MATLAB Function : MATLAB Function  TreatAsAtomicUnit=on
  Out1 : Outport
  wires:
  In1/1 -> Data Type Conversion/1
  Data Type Conversion1/1 -> MATLAB Function/2(prevData)
  Data Type Conversion/1 -> MATLAB Function/1(inData)
  Delay/1 -> Data Type Conversion1/1
  MATLAB Function/1(inData_Output) -> Out1/1, Delay/1
  Delay1/1 -> MATLAB Function/3(Error)
  MATLAB Function/2(Error_Last) -> Delay1/1

== system Demo919/Function-Call Subsystem1/Torque_Control/Kalman_Filer3 ==
  In1 : Inport
  Data Type Conversion : DataTypeConversion  OutDataTypeStr=single
  Data Type Conversion1 : DataTypeConversion  OutDataTypeStr=single
  Delay : Delay  DelayLength=1  InitialCondition=0
  Delay1 : Delay  DelayLength=1  InitialCondition=0
  MATLAB Function : MATLAB Function  TreatAsAtomicUnit=on
  Out1 : Outport
  wires:
  MATLAB Function/2(Error_Last) -> Delay1/1
  Delay1/1 -> MATLAB Function/3(Error)
  MATLAB Function/1(inData_Output) -> Delay/1, Out1/1
  Delay/1 -> Data Type Conversion1/1
  Data Type Conversion/1 -> MATLAB Function/1(inData)
  Data Type Conversion1/1 -> MATLAB Function/2(prevData)
  In1/1 -> Data Type Conversion/1

== system Demo919/Function-Call Subsystem1/Torque_Control/Kalman_Filer4 ==
  In1 : Inport
  Data Type Conversion : DataTypeConversion  OutDataTypeStr=single
  Data Type Conversion1 : DataTypeConversion  OutDataTypeStr=single
  Delay : Delay  DelayLength=1  InitialCondition=0
  Delay1 : Delay  DelayLength=1  InitialCondition=0
  MATLAB Function : MATLAB Function  TreatAsAtomicUnit=on
  Out1 : Outport
  wires:
  In1/1 -> Data Type Conversion/1
  Data Type Conversion1/1 -> MATLAB Function/2(prevData)
  Data Type Conversion/1 -> MATLAB Function/1(inData)
  Delay/1 -> Data Type Conversion1/1
  MATLAB Function/1(inData_Output) -> Out1/1, Delay/1
  Delay1/1 -> MATLAB Function/3(Error)
  MATLAB Function/2(Error_Last) -> Delay1/1

== system Demo919/Function-Call Subsystem1/Torque_Control/OQ2 ==
  In1 : Inport  OutMin=0  OutMax=10000
  Bitwise Operator : simulink/Logic and Bit Operations/Bitwise Operator  logicop=AND  UseBitMask=on  BitMask=bin2dec('11111111')  BitMaskRealWorld=Stored Integer
  Data Type Conversion : DataTypeConversion  OutDataTypeStr=uint8
  Data Type Conversion1 : DataTypeConversion  OutDataTypeStr=uint8
  Shift Arithmetic : ArithShift  BitShiftNumber=8  BitShiftDirection=Right
  Mot_SpeedH : Outport
  Mot_SpeedL : Outport  Port=2
  wires:
  Shift Arithmetic/1 -> Data Type Conversion/1
  Data Type Conversion/1 -> Mot_SpeedH/1
  Bitwise Operator/1 -> Data Type Conversion1/1
  Data Type Conversion1/1 -> Mot_SpeedL/1
  In1/1 -> Bitwise Operator/1, Shift Arithmetic/1

== system Demo919/Function-Call Subsystem1/Torque_Control/OQ3 ==
  In1 : Inport  OutMin=0  OutMax=10000
  Bitwise Operator : simulink/Logic and Bit Operations/Bitwise Operator  logicop=AND  UseBitMask=on  BitMask=bin2dec('11111111')  BitMaskRealWorld=Stored Integer
  Data Type Conversion : DataTypeConversion  OutDataTypeStr=uint8
  Data Type Conversion1 : DataTypeConversion  OutDataTypeStr=uint8
  Shift Arithmetic : ArithShift  BitShiftNumber=8  BitShiftDirection=Right
  Mot_SpeedH : Outport
  Mot_SpeedL : Outport  Port=2
  wires:
  Shift Arithmetic/1 -> Data Type Conversion/1
  Data Type Conversion/1 -> Mot_SpeedH/1
  Bitwise Operator/1 -> Data Type Conversion1/1
  Data Type Conversion1/1 -> Mot_SpeedL/1
  In1/1 -> Bitwise Operator/1, Shift Arithmetic/1

== system Demo919/Function-Call Subsystem1/Torque_Control/Subsystem ==
  In1 : Inport
  In2 : Inport  Port=2
  In3 : Inport  Port=3
  In4 : Inport  Port=4
  Add{,1..4} (5 alike) : Sum
  Data Type Conversion5 : DataTypeConversion  OutDataTypeStr=double
  Data Type Conversion6 : DataTypeConversion  OutDataTypeStr=double
  Gain : Gain  Gain=0.5
  Gain3 : Gain  Gain=0.5
  Gain4 : Gain  Gain=0.5
  PID Controller : simulink/Continuous/PID Controller  Controller=PI  Form=Parallel  TimeDomain=Discrete-time  SampleTime=-1  IntegratorMethod=Forward Euler  FilterMethod=Forward Euler  ControllerParametersSource=internal  P=8  I=0.0001  D=0  UseFilter=on  N=100  TunerSelectOption=Transfer Function Based (PID Tuner App)  InitialConditionSource=internal  InitialConditionForIntegrator=0  InitialConditionForFilter=0  DifferentiatorICPrevScaledInput=0  ExternalReset=none  TrackingMode=off  Kt=1  LimitOutput=off  UpperSaturationLimit=inf  LowerSaturationLimit=-inf  LinearizeAsGain=on  AntiWindupMode=none  Kb=1  POutMin=[]  POutMax=[]  IOutMin=[]  IOutMax=[]  DOutMin=[]  DOutMax=[]  NOutMin=[]  NOutMax=[]  SumOutMin=[]  SumOutMax=[]  SaturationOutMin=[]  SaturationOutMax=[]  PParamMin=[]  PParamMax=[]  IParamMin=[]  IParamMax=[]  DParamMin=[]  DParamMax=[]  NParamMin=[]  NParamMax=[]  KbParamMin=[]  KbParamMax=[]  KtParamMin=[]  KtParamMax=[]  KbOutMin=[]  KbOutMax=[]  KtOutMin=[]  KtOutMax=[]  IntegratorOutMin=[]  IntegratorOutMax=[]  FilterOutMin=[]  FilterOutMax=[]  SumI1OutMin=[]  SumI1OutMax=[]  SumI2OutMin=[]  SumI2OutMax=[]  SumI3OutMin=[]  SumI3OutMax=[]  SumI4OutMin=[]  SumI4OutMax=[]  SumDOutMin=[]  SumDOutMax=[]  DifferentiatorOutMin=[]  DifferentiatorOutMax=[]  FilterDiffOutCoefMin=[]  FilterDiffOutCoefMax=[]  ReciprocalOutMin=[]  ReciprocalOutMax=[]  SumDenOutMin=[]  SumDenOutMax=[]  SumNumOutMin=[]  SumNumOutMax=[]  DivideOutMin=[]  DivideOutMax=[]  IntegratorContinuousStateAttributes=''  IntegratorStateMustResolveToSignalObject=off  IntegratorRTWStateStorageClass=Auto  FilterContinuousStateAttributes=''  FilterStateMustResolveToSignalObject=off  FilterRTWStateStorageClass=Auto  ParallelPVariant=InternalParameters  IdealPVariant=Disabled  IVariant=InternalParameters  DVariant=Disabled  IntegratorVariant=Discrete  SatVariant=Disabled  AWVariant=Passthrough  PCopyVariant=Disabled  TRVariant=Disabled  FdbkBlocksVariant=Forward  IdealPFdbkVariant=Disabled  SatFdbkVariant=Disabled  DerivativeFilterVariant=Disabled  NVariant=Disabled  NCopyVariant=Disabled_SignalSpec  FilterICVariant=Disabled  IntegratorICVariant=InternalICs  ExternalResetVariant=Disabled  TRSumVariant=Passthrough  SumFdbkVariant=Disabled  SumVariant=Sum_PI
  PID Controller1 : simulink/Continuous/PID Controller  Controller=PI  Form=Parallel  TimeDomain=Discrete-time  SampleTime=-1  IntegratorMethod=Forward Euler  FilterMethod=Forward Euler  ControllerParametersSource=internal  P=8  I=0.0001  D=0  UseFilter=on  N=100  TunerSelectOption=Transfer Function Based (PID Tuner App)  InitialConditionSource=internal  InitialConditionForIntegrator=0  InitialConditionForFilter=0  DifferentiatorICPrevScaledInput=0  ExternalReset=none  TrackingMode=off  Kt=1  LimitOutput=off  UpperSaturationLimit=inf  LowerSaturationLimit=-inf  LinearizeAsGain=on  AntiWindupMode=none  Kb=1  POutMin=[]  POutMax=[]  IOutMin=[]  IOutMax=[]  DOutMin=[]  DOutMax=[]  NOutMin=[]  NOutMax=[]  SumOutMin=[]  SumOutMax=[]  SaturationOutMin=[]  SaturationOutMax=[]  PParamMin=[]  PParamMax=[]  IParamMin=[]  IParamMax=[]  DParamMin=[]  DParamMax=[]  NParamMin=[]  NParamMax=[]  KbParamMin=[]  KbParamMax=[]  KtParamMin=[]  KtParamMax=[]  KbOutMin=[]  KbOutMax=[]  KtOutMin=[]  KtOutMax=[]  IntegratorOutMin=[]  IntegratorOutMax=[]  FilterOutMin=[]  FilterOutMax=[]  SumI1OutMin=[]  SumI1OutMax=[]  SumI2OutMin=[]  SumI2OutMax=[]  SumI3OutMin=[]  SumI3OutMax=[]  SumI4OutMin=[]  SumI4OutMax=[]  SumDOutMin=[]  SumDOutMax=[]  DifferentiatorOutMin=[]  DifferentiatorOutMax=[]  FilterDiffOutCoefMin=[]  FilterDiffOutCoefMax=[]  ReciprocalOutMin=[]  ReciprocalOutMax=[]  SumDenOutMin=[]  SumDenOutMax=[]  SumNumOutMin=[]  SumNumOutMax=[]  DivideOutMin=[]  DivideOutMax=[]  IntegratorContinuousStateAttributes=''  IntegratorStateMustResolveToSignalObject=off  IntegratorRTWStateStorageClass=Auto  FilterContinuousStateAttributes=''  FilterStateMustResolveToSignalObject=off  FilterRTWStateStorageClass=Auto  ParallelPVariant=InternalParameters  IdealPVariant=Disabled  IVariant=InternalParameters  DVariant=Disabled  IntegratorVariant=Discrete  SatVariant=Disabled  AWVariant=Passthrough  PCopyVariant=Disabled  TRVariant=Disabled  FdbkBlocksVariant=Forward  IdealPFdbkVariant=Disabled  SatFdbkVariant=Disabled  DerivativeFilterVariant=Disabled  NVariant=Disabled  NCopyVariant=Disabled_SignalSpec  FilterICVariant=Disabled  IntegratorICVariant=InternalICs  ExternalResetVariant=Disabled  TRSumVariant=Passthrough  SumFdbkVariant=Disabled  SumVariant=Sum_PI
  Saturation2 : Saturate  UpperLimit=6000  LowerLimit=0  OutDataTypeStr=double
  Saturation3 : Saturate  UpperLimit=6000  LowerLimit=0  OutDataTypeStr=double
  Sum1 : Sum  Inputs=|+-
  Sum2 : Sum  Inputs=|+-
  Out1 : Outport
  Out2 : Outport  Port=2
  wires:
  PID Controller1/1 -> Saturation3/1
  Add1/1 -> PID Controller1/1
  Sum2/1 -> Add/2
  Add2/1 -> Gain/1
  In4/1 -> Data Type Conversion6/1
  Data Type Conversion5/1 -> Sum2/2
  In1/1 -> Add2/2, Add3/1, Sum2/1
  Add3/1 -> Gain3/1
  Gain3/1 -> Add/1
  In2/1 -> Data Type Conversion5/1
  Sum1/1 -> Add1/1
  Add/1 -> PID Controller/1
  PID Controller/1 -> Saturation2/1
  In3/1 -> Add2/1, Add4/2, Sum1/1
  Data Type Conversion6/1 -> Sum1/2
  Gain4/1 -> Add1/2
  Gain/1 -> Add4/1, Add3/2
  Add4/1 -> Gain4/1
  Saturation3/1 -> Out2/1
  Saturation2/1 -> Out1/1

== system Demo919/Function-Call Subsystem1/Torque_Control/Subsystem1 ==
  "Brake " : Inport
  L_Pri : Inport  Port=2
  L_Maped : Inport  Port=3
  R_Pri : Inport  Port=4
  R_Maped : Inport  Port=5
  AcPed_Reliable : Stateflow chart  Commented=on  TreatAsAtomicUnit=on
  AcPed_Reliable1 : Stateflow chart  TreatAsAtomicUnit=on
  AcPed_Reliable2 : Stateflow chart  Commented=on  TreatAsAtomicUnit=on
  AcPed_Reliable3 : Stateflow chart  TreatAsAtomicUnit=on
  Ac_Arbitrate : Stateflow chart  TreatAsAtomicUnit=on
  MeaModule10 : ec5744lib/RapidECU_U3/07Calibration/MeaModule  signal=Pedal_trH
      settings: SourceProductName=ECUCoder for MPC5744
  Subsystem : Subsystem
  "pedal_tr " : Outport
  "Pedal_WS " : Outport  Port=2
  wires:
  R_Pri/1 -> AcPed_Reliable3/1(Pedal_TrL), AcPed_Reliable/1(Pedal_TrL), AcPed_Reliable2/1(Pedal_TrL)
  AcPed_Reliable1/1(Pedal_WrongState) -> Subsystem/2(Pedal_Ws2)
  MeaModule10/1 -> Ac_Arbitrate/1(Pedal_TrH)
  Ac_Arbitrate/1(Pedal_Tr) -> Subsystem/3(Pedal_Tr)
  "Brake "/1 -> AcPed_Reliable1/1(Brake)
  R_Maped/1 -> Ac_Arbitrate/2(Pedal_TrL)
  L_Pri/1 -> AcPed_Reliable3/2(Pedal_TrH), AcPed_Reliable/2(Pedal_TrH), AcPed_Reliable2/2(Pedal_TrH)
  L_Maped/1 -> MeaModule10/1
  Subsystem/1(Out1) -> "pedal_tr "/1
  Subsystem/2(Pedal_WS) -> "Pedal_WS "/1
  AcPed_Reliable3/1(Pedal_WrongState) -> Subsystem/1(Pedal_WS1)
